simulink model "Linealidad"  (R2023b)
settings: Solver=VariableStepAuto  StartTime=0.0  StopTime=10.0  RelTol=1e-3
settings Model: Creator=diavl  LastModifiedBy=diavl

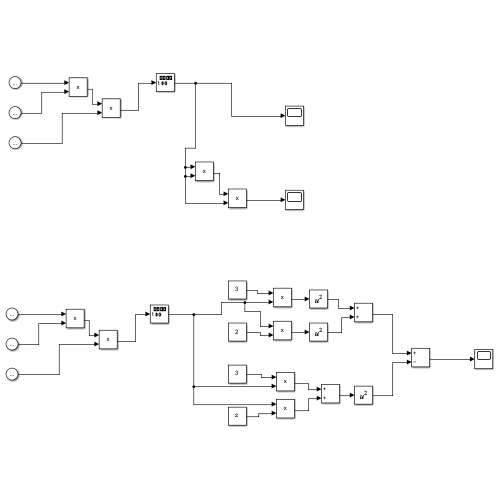
[thumbnail: Simulink's stored preview of the top-level diagram]
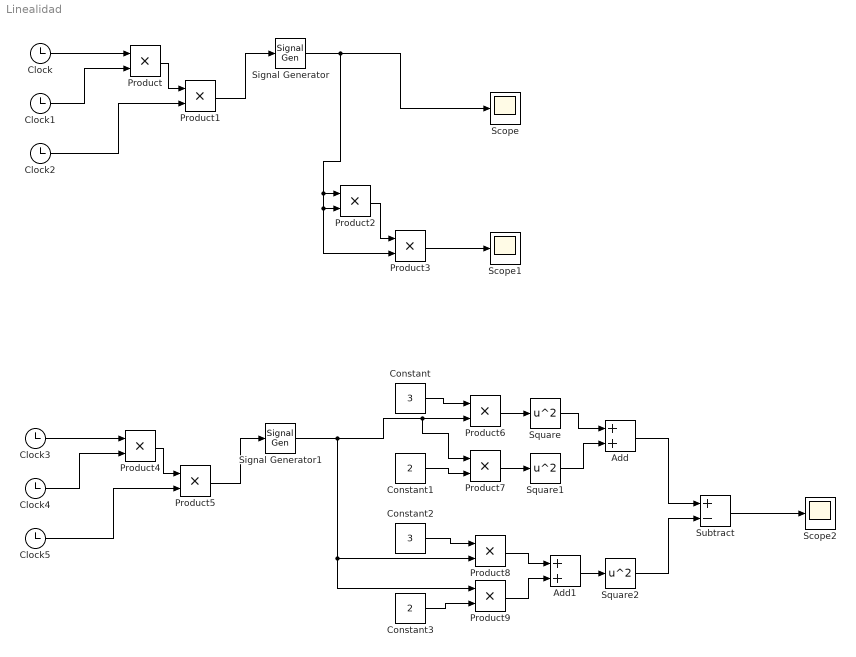
== system Linealidad ==
  Add : Sum
  Add1 : Sum
  Clock{,1..5} (6 alike) : Clock
  Constant : Constant  Value=3
  Constant1 : Constant  Value=2
  Constant2 : Constant  Value=3
  Constant3 : Constant  Value=2
  Product{,1..9} (10 alike) : Product
  Scope : Scope
  Scope1 : Scope
  Scope2 : Scope
  Signal Generator : SignalGenerator  TimeSource=Use external signal  Frequency=10
  Signal Generator1 : SignalGenerator  TimeSource=Use external signal  Frequency=10
  Square : Math  Operator=square
  Square1 : Math  Operator=square
  Square2 : Math  Operator=square
  Subtract : Sum  Inputs=+-
  wires:
  Signal Generator/1 -> Product3/2, Product2/2, Product2/1, Scope/1
  Product1/1 -> Signal Generator/1
  Product/1 -> Product1/1
  Clock/1 -> Product/1
  Clock2/1 -> Product1/2
  Clock1/1 -> Product/2
  Product2/1 -> Product3/1
  Product3/1 -> Scope1/1
  Clock4/1 -> Product4/2
  Clock3/1 -> Product4/1
  Product5/1 -> Signal Generator1/1
  Clock5/1 -> Product5/2
  Product4/1 -> Product5/1
  Constant/1 -> Product6/1
  Signal Generator1/1 -> Product9/1, Product8/2, Product7/1, Product6/2
  Constant1/1 -> Product7/2
  Product6/1 -> Square/1
  Product7/1 -> Square1/1
  Square/1 -> Add/1
  Square1/1 -> Add/2
  Constant3/1 -> Product9/2
  Constant2/1 -> Product8/1
  Product8/1 -> Add1/1
  Product9/1 -> Add1/2
  Add1/1 -> Square2/1
  Add/1 -> Subtract/1
  Square2/1 -> Subtract/2
  Subtract/1 -> Scope2/1
